simulink model "LAB3_Linear"  (R2025b)
settings: Solver=VariableStepAuto  StartTime=0.0  StopTime=10.0  RelTol=1e-3
libraries: simulink x1
settings Model: Creator=Wingshingsho  LastModifiedBy=Wingshingsho

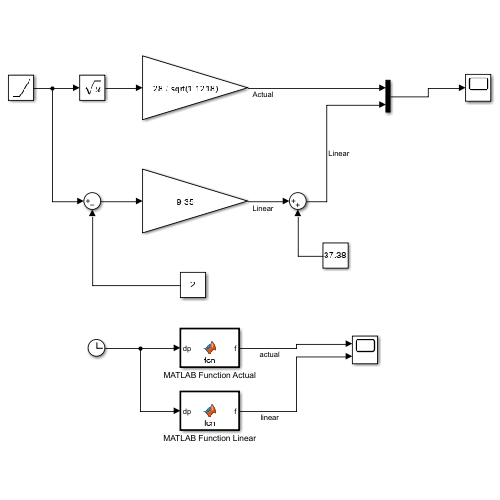
[thumbnail: Simulink's stored preview of the top-level diagram]
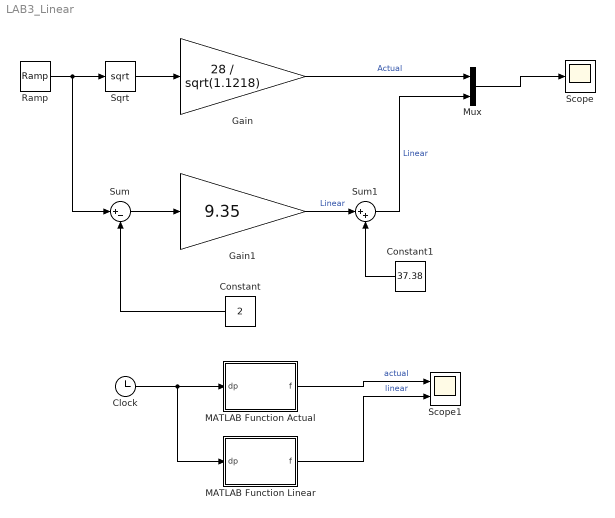
== system LAB3_Linear ==
  Clock : Clock
  Constant : Constant  Value=2
  Constant1 : Constant  Value=37.38
  Gain : Gain  Gain=28 / sqrt(1.1218)
  Gain1 : Gain  Gain=9.35
  MATLAB Function Actual : MATLAB Function  TreatAsAtomicUnit=on
  MATLAB Function Linear : MATLAB Function  TreatAsAtomicUnit=on
  Mux : Mux  Inputs=2
  Ramp : simulink/Sources/Ramp  slope=1  start=0  InitialOutput=0
  Scope : Scope
      settings: ActiveDisplayYMinimum=-4.7035882047915081  ActiveDisplayYMaximum=110.65986632290013
  Scope1 : Scope  NumInputPorts=2
      settings: ActiveDisplayYMinimum=-16.937660455936985  ActiveDisplayYMaximum=137.66040204406312
  Sqrt : Sqrt
  Sum : Sum  Inputs=|+-
  Sum1 : Sum  Inputs=|++
  wires:
  Ramp/1 -> Sum/1, Sqrt/1
  Sqrt/1 -> Gain/1
  Mux/1 -> Scope/1
  Gain/1 -> Mux/1  "Actual"
  Sum/1 -> Gain1/1
  Constant/1 -> Sum/2
  Gain1/1 -> Sum1/1  "Linear"
  Constant1/1 -> Sum1/2
  Sum1/1 -> Mux/2  "Linear"
  Clock/1 -> MATLAB Function Linear/1(dp), MATLAB Function Actual/1(dp)
  MATLAB Function Actual/1(f) -> Scope1/1  "actual"
  MATLAB Function Linear/1(f) -> Scope1/2  "linear"

== matlab function LAB3_Linear/MATLAB Function Actual ==
  data: dp input; f output
function f = fcn(dp)

f = 28*sqrt(dp/(70/62.4)) ;

end

== matlab function LAB3_Linear/MATLAB Function Linear ==
  data: dp input; f output
function f = fcn(dp)

f = 37.386 + 9.3466*(dp-2);

end
